simulink model "DAS"  (R2012b)
settings: Solver=FixedStepDiscrete  StartTime=0.0  StopTime=inf  FixedStep=0.1  RelTol=1e-3
PreLoadFcn:
  | if exist('tl_preloadfcn','file'), tl_preloadfcn(gcs,101); end
PostLoadFcn:
  | if exist('tl_postloadfcn','file'), tl_postloadfcn(gcs,101); end
InitFcn:
  | if exist('tlds_init','file'), tlds_init(gcs); end
StartFcn:
  | if exist('tlds_start','file'), tlds_start(gcs); end
StopFcn:
  | if exist('tlds_stop','file'), tlds_stop(gcs); end
undefined symbols (not defined in the file): A, B, C, Dd, DEMO_FAS_Accusti_Threshold_Time, DEMO_FAS_BrakeBooster_Threshold, DEMO_FAS_CC_DELTA, DEMO_FAS_CC_Lvl2_Round, DEMO_FAS_CC_Min_Value, DEMO_FAS_Distance_Treshold_Far, DEMO_FAS_Distance_Treshold_Med, DEMO_FAS_Distance_Treshold_Near, DEMO_FAS_Distronic, DEMO_FAS_Emerg_Brake_Force1, DEMO_FAS_Emerg_Brake_Force2, DEMO_FAS_Emerg_Brake_Time1, DEMO_FAS_Emerg_Brake_Time2, DEMO_FAS_EmergencyBrake, DEMO_FAS_FollowToStop, DEMO_FAS_Limiter, DEMO_FAS_Limiter_DELTA, DEMO_FAS_Neg_Max_ms, DEMO_FAS_Opti_Threshold_Time, DEMO_FAS_Repeater, DEMO_FAS_Repeater_Time, DEMO_FAS_Signdetection, DEMO_FAS_Tempomat
(part 7 of 11)

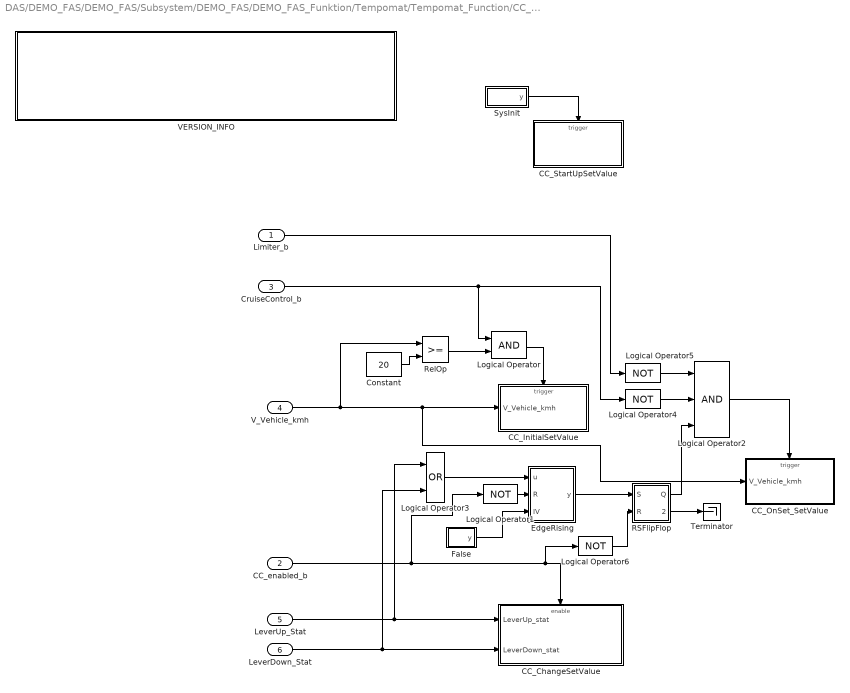
== system DAS/DEMO_FAS/DEMO_FAS/Subsystem/DEMO_FAS/DEMO_FAS_Funktion/Tempomat/Tempomat_Function/CC_SetValue ==
  Limiter_b : Inport
  CC_enabled_b : Inport  Port=2
  CruiseControl_b : Inport  Port=3
  V_Vehicle_kmh : Inport  Port=4
  LeverUp_Stat : Inport  Port=5
  LeverDown_Stat : Inport  Port=6
  CC_ChangeSetValue : Subsystem  TreatAsAtomicUnit=on
  CC_InitialSetValue : Subsystem  TreatAsAtomicUnit=on
  CC_OnSet_SetValue : Subsystem  TreatAsAtomicUnit=on
  CC_StartUpSetValue : Subsystem  TreatAsAtomicUnit=on
  Constant : Constant  Value=20  mask(TL_Constant){data={'date',735343.57031072921}}
      settings: CopyFcn=if exist('tl_reset_reviewflag') == 2, tl_reset_reviewflag(gcbh); end  DeleteFcn=if exist('delete_tlblock','file')==2,delete_tlblock(gcbh);end  NameChangeFcn=if exist('rename_tlblock','file')==2,rename_tlblock(gcbh);end  OpenFcn=if exist('tl_open_blockdlg','file')==2,tl_open_blockdlg(gcbh);else,open_system(gcbh,'parameter');end
      mask Help: eval(['if exist(''tl_online_help'',''file'') == 2, tl_online_help(''Topic'',''TL_Constant''),else, web([''jar:file:///'',matlabroot,''/help/toolbox/simulink/help.jar!/slref/' lower(get_param(gcbh,'Blocktype')) '.html''], ''-helpbrowser''),end'])
      mask Display: plot([-0.05, 1.05, NaN, -0.05, 1.05],[.01, .01, NaN, .99, .99])
  EdgeRising : Subsystem  mask(TLMSR_V200_EdgeRising){dT=-1, YName=}
      mask prompts: dT "Sampe Time"; YName "Y OutName"
      mask help:
      | The output indicates TRUE if the input value changes from FALSE to TRUE.
      | Reset input 'R' on TRUE will write the initial value 'IV' to the internal memory.
      mask init:
      | % TL block lines
      | x1=[0 0 1 1 0];
      | y1=[1 0 0 1 1];
      | x2=[1 0];
      | y2=[.96 .96];
      | x3=[0 1];
      | y3=[.04 .04];
      | 
      | tl_act_sg_init_blk;
      mask Help:
      | <HTML>
      | <HEAD>
      | <META HTTP-EQUIV="Content-Type" CONTENT="text/html; charset=iso-8859-1">
      | <TITLE>Help</TITLE>
      | </HEAD>
      | <BODY>
      | 
      | <B><FONT FACE="Arial"><P>Function:</P>
      | </B><P>The block detects a rising edge of the logical input signal <FONT FACE="Courier New">u</FONT> and indicates this change at the output <FONT FACE="Courier New">y</FONT> for one cycle.</P>
      | 
      | <B><P>In-/Outputs:</P>
      | </B>
      | <P><U>Input</U></P>
      | <P>The block input </FONT><FONT FACE="Courier New">u</FONT><FONT FACE="Arial"> must be connected to the input signal.</P>
      | 
      | <U><P>Reset / Initial Value</P>
      | </U><P>If the reset input </FONT><FONT FACE="Courier New">R</FONT><FONT FACE="Arial"> gets a '1' signal the block will write the initial value <FONT FACE="Courier New">IV</FONT> to its internal memory. A logical '1' at <FONT FACE="Courier New">IV</FONT>
      | will prevent the output to become TRUE during reset.</P>
      | 
      | <U><P>Output</P>
      | </U><P>The output </FONT><FONT FACE="Courier New">y</FONT><FONT FACE="Arial"> shows '1' if a rising edge at the input signal <FONT FACE="Courier New">u</FONT> is detected.</P>
      | </FONT></BODY>
      | </HTML>
      mask Display:
      | plot(x1,y1,x2,y2,x3,y3);
      | image(imread('EdgeRising.tif','tif'),[0.25,0.2,0.5,0.6])
  False : Subsystem  mask(TLACT_SG_V200_False){}
      mask help: False
      mask init:
      | % TL block lines
      | x1=[0 0 1 1 0];
      | y1=[1 0 0 1 1];
      | x2=[1 0];
      | y2=[.9 .9];
      | x3=[0 1];
      | y3=[.1 .1];
      settings: OpenFcn=open_system([gcb, '/Zero'], 'OpenFcn')
      mask Display:
      | plot(x1,y1,x2,y2,x3,y3);
      | disp('False');
  Logical Operator : Logic  AllPortsSameDT=off  OutDataTypeStr=boolean  mask(TL_LogicalOperator){data={'date',735343.57067486108}}
      settings: DeleteFcn=if exist('delete_tlblock','file')==2,delete_tlblock(gcbh);end  NameChangeFcn=if exist('rename_tlblock','file')==2,rename_tlblock(gcbh);end  OpenFcn=if exist('tl_open_blockdlg','file')==2,tl_open_blockdlg(gcbh);else,open_system(gcbh,'parameter');end
      mask Help: eval(['if exist(''tl_online_help'',''file'') == 2, tl_online_help(''Topic'',''TL_LogicalOperator''),else, web([''jar:file:///'',matlabroot,''/help/toolbox/simulink/help.jar!/slref/' lower(get_param(gcbh,'Blocktype')) '.html''], ''-helpbrowser''),end'])
      mask Display: plot([-0.05, 1.05, NaN, -0.05, 1.05],[.01, .01, NaN, .99, .99])
  Logical Operator{1,4..6} (4 alike) : Logic  Operator=NOT  Inputs=1  AllPortsSameDT=off  OutDataTypeStr=boolean  mask(TL_LogicalOperator){data={'date',735346.37280901615}}
      settings: DeleteFcn=if exist('delete_tlblock','file')==2,delete_tlblock(gcbh);end  NameChangeFcn=if exist('rename_tlblock','file')==2,rename_tlblock(gcbh);end  OpenFcn=if exist('tl_open_blockdlg','file')==2,tl_open_blockdlg(gcbh);else,open_system(gcbh,'parameter');end
      mask Help: eval(['if exist(''tl_online_help'',''file'') == 2, tl_online_help(''Topic'',''TL_LogicalOperator''),else, web([''jar:file:///'',matlabroot,''/help/toolbox/simulink/help.jar!/slref/' lower(get_param(gcbh,'Blocktype')) '.html''], ''-helpbrowser''),end'])
      mask Display: plot([-0.05, 1.05, NaN, -0.05, 1.05],[.01, .01, NaN, .99, .99])
  Logical Operator2 : Logic  Inputs=3  AllPortsSameDT=off  OutDataTypeStr=boolean  mask(TL_LogicalOperator){data={'date',735346.47148690966}}
      settings: DeleteFcn=if exist('delete_tlblock','file')==2,delete_tlblock(gcbh);end  NameChangeFcn=if exist('rename_tlblock','file')==2,rename_tlblock(gcbh);end  OpenFcn=if exist('tl_open_blockdlg','file')==2,tl_open_blockdlg(gcbh);else,open_system(gcbh,'parameter');end
      mask Help: eval(['if exist(''tl_online_help'',''file'') == 2, tl_online_help(''Topic'',''TL_LogicalOperator''),else, web([''jar:file:///'',matlabroot,''/help/toolbox/simulink/help.jar!/slref/' lower(get_param(gcbh,'Blocktype')) '.html''], ''-helpbrowser''),end'])
      mask Display: plot([-0.05, 1.05, NaN, -0.05, 1.05],[.01, .01, NaN, .99, .99])
  Logical Operator3 : Logic  Operator=OR  AllPortsSameDT=off  OutDataTypeStr=boolean  mask(TL_LogicalOperator){data={'date',735346.37234638887}}
      settings: DeleteFcn=if exist('delete_tlblock','file')==2,delete_tlblock(gcbh);end  NameChangeFcn=if exist('rename_tlblock','file')==2,rename_tlblock(gcbh);end  OpenFcn=if exist('tl_open_blockdlg','file')==2,tl_open_blockdlg(gcbh);else,open_system(gcbh,'parameter');end
      mask Help: eval(['if exist(''tl_online_help'',''file'') == 2, tl_online_help(''Topic'',''TL_LogicalOperator''),else, web([''jar:file:///'',matlabroot,''/help/toolbox/simulink/help.jar!/slref/' lower(get_param(gcbh,'Blocktype')) '.html''], ''-helpbrowser''),end'])
      mask Display: plot([-0.05, 1.05, NaN, -0.05, 1.05],[.01, .01, NaN, .99, .99])
  RSFlipFlop : Subsystem  mask(TLMSR_V200_RSFlipFlop){dT=-1, QName=, QNName=}
      mask prompts: dT "SampleTime"; QName "Q OutName"; QNName "QN OutName"
      mask help: A flip flop. The 'R' input (reset) dominates the 'S' input (set).
      mask init:
      | % TL block lines
      | x1=[0 0 1 1 0];
      | y1=[1 0 0 1 1];
      | x2=[1 0];
      | y2=[.96 .96];
      | x3=[0 1];
      | y3=[.04 .04];
      | 
      | tl_act_sg_init_blk;
      mask Help:
      | <HTML>
      | <HEAD>
      | <META HTTP-EQUIV="Content-Type" CONTENT="text/html; charset=iso-8859-1">
      | <TITLE>test</TITLE>
      | </HEAD>
      | 
      | <B><FONT FACE="Arial"><P>Function:</P>
      | </B><P>The block provides the function of a RS-Flip-Flop with the reset input </FONT><FONT FACE="Courier New">R</FONT><FONT FACE="Arial"> dominating over the set input </FONT><FONT FACE="Courier New">S</FONT><FONT FACE="Arial">. An inverted output </FONT><FONT FACE="Courier New">/Q</FONT><FONT FACE="Arial"> is provided.</P>
      | </FONT>
      | <TABLE BORDER CELLSPACING=1 CELLPADDING=4 WIDTH=506>
      | <TR><TD WIDTH="25%" VALIGN="TOP">
      | <B><FONT FACE="Arial"><P ALIGN="CENTER">S</B></FONT></TD>
      | <TD WIDTH="25%" VALIGN="TOP">
      | <B><FONT FACE="Arial"><P ALIGN="CENTER">R</B></FONT></TD>
      | <TD WIDTH="25%" VALIGN="TOP">
      | <B><FONT FACE="Arial"><P ALIGN="CENTER">Q</B></FONT></TD>
      | <TD WIDTH="25%" VALIGN="TOP">
      | <B><FONT FACE="Arial"><P ALIGN="CENTER">/Q</B></FONT></TD>
      | </TR>
      | <TR><TD WIDTH="25%" VALIGN="TOP">
      | <FONT FACE="Arial"><P ALIGN="CENTER">0</FONT></TD>
      | <TD WIDTH="25%" VALIGN="TOP">
      | <FONT FACE="Arial"><P ALIGN="CENTER">0</FONT></TD>
      | <TD WIDTH="25%" VALIGN="TOP">
      | <FONT FACE="Arial"><P ALIGN="CENTER">Q(n-1)</FONT></TD>
      | <TD WIDTH="25%" VALIGN="TOP">
      | <FONT FACE="Arial"><P ALIGN="CENTER">/Q(n-1)</FONT></TD>
      | </TR>
      | <TR><TD WIDTH="25%" VALIGN="TOP">
      | <FONT FACE="Arial"><P ALIGN="CENTER">0</FONT></TD>
      | <TD WIDTH="25%" VALIGN="TOP">
      | <FONT FACE="Arial"><P ALIGN="CENTER">1</FONT></TD>
      | <TD WIDTH="25%" VALIGN="TOP">
      | <FONT FACE="Arial"><P ALIGN="CENTER">0</FONT></TD>
      | <TD WIDTH="25%" VALIGN="TOP">
      | <FONT FACE="Arial"><P ALIGN="CENTER">1</FONT></TD>
      | </TR>
      | <TR><TD WIDTH="25%" VALIGN="TOP">
      | <FONT FACE="Arial"><P ALIGN="CENTER">1</FONT></TD>
      | <TD WIDTH="25%" VALIGN="TOP">
      | <FONT FACE="Arial"><P ALIGN="CENTER">0</FONT></TD>
      | <TD WIDTH="25%" VALIGN="TOP">
      | <FONT FACE="Arial"><P ALIGN="CENTER">1</FONT></TD>
      | <TD WIDTH="25%" VALIGN="TOP">
      | <FONT FACE="Arial"><P ALIGN="CENTER">0</FONT></TD>
      | </TR>
      | <TR><TD WIDTH="25%" VALIGN="TOP">
      | <FONT FACE="Arial"><P ALIGN="CENTER">1</FONT></TD>
      | <TD WIDTH="25%" VALIGN="TOP">
      | <FONT FACE="Arial"><P ALIGN="CENTER">1</FONT></TD>
      | <TD WIDTH="25%" VALIGN="TOP">
      | <FONT FACE="Arial"><P ALIGN="CENTER">0</FONT></TD>
      | <TD WIDTH="25%" VALIGN="TOP">
      | <FONT FACE="Arial"><P ALIGN="CENTER">1</FONT></TD>
      | </TR>
      | </TABLE>
      | 
      | <FONT FACE="Arial">
      | <B><P>In-/Outputs:</P>
      | </B><U><P>S</P>
      | </U><P>The set input </FONT><FONT FACE="Courier New">S</FONT><FONT FACE="Arial"> on '1' will set the output </FONT><FONT FACE="Courier New">Q</FONT><FONT FACE="Arial"> if the reset input </FONT><FONT FACE="Courier New">R</FONT><FONT FACE="Arial"> is '0'.</P>
      | <U><P>R</P>
      | </U><P>The reset input </FONT><FONT FACE="Courier New">R</FONT><FONT FACE="Arial"> on '1' will reset the output </FONT><FONT FACE="Courier New">Q</FONT><FONT FACE="Arial">.</P>
      | <U><P>Q, /Q</P>
      | </U><P>The output </FONT><FONT FACE="Courier New">Q</FONT><FONT FACE="Arial"> shows the state of the internal memory. </FONT><FONT FACE="Courier New">/Q</FONT><FONT FACE="Arial"> contains the inverted state of </FONT><FONT FACE="Courier New">Q</FONT><FONT FACE="Arial">.</P></FONT>
      | </HTML>
      mask Display:
      | plot(x1,y1,x2,y2,x3,y3);
      | image(imread('RSFlipFlop.tif','tif'),[0.05,0.1,0.9,0.8])
  RelOp : RelationalOperator  Description=|  mask(TL_RelationalOperator){data={'logdata',{'plotchannels',[]},'date',735343.572069132}}
      | Relational operator block of dSPACE TargetLink.
      | 
      | This block performs a relational operation on its two inputs u1 and u2 and produces output according to the following table.
      | If the result is TRUE, the output is 1; if FALSE, it is 0.
      | 
      | Operator   Output
      |  ==        TRUE if u1 is equal to u2
      |  !=        TRUE if u1 is not equal to u2
      |  <         TRUE if u1 is less than u2
      |  <=        TRUE if u1 is less than or equal to u2
      |  >=        TRUE if u1 is greater than or equal to u2
      |  >         TRUE if u1 is greater than u2
      settings: DeleteFcn=if exist('delete_tlblock','file')==2,delete_tlblock(gcbh);end  NameChangeFcn=if exist('rename_tlblock','file')==2,rename_tlblock(gcbh);end  OpenFcn=if exist('tl_open_blockdlg','file')==2,tl_open_blockdlg(gcbh);else,open_system(gcbh,'parameter');end
      mask Help: eval(['if exist(''tl_online_help'',''file'') == 2, tl_online_help(''Topic'',''TL_RelationalOperator''),else, web([''jar:file:///'',matlabroot,''/help/toolbox/simulink/help.jar!/slref/' lower(get_param(gcbh,'Blocktype')) '.html''], ''-helpbrowser''),end'])
      mask Display: plot([-0.05, 1.05, NaN, -0.05, 1.05],[.01, .01, NaN, .99, .99])
  SysInit : Subsystem  mask(TLACT_SG_V200_SysInit){dT=-1, YName=}
      mask prompts: dT "Sample Time"; YName "Y OutName"
      mask help: An inital pulse is generated for for the first block evaluation.
      mask init:
      | % TL block lines
      | x1=[0 0 1 1 0];
      | y1=[1 0 0 1 1];
      | x2=[1 0];
      | y2=[.92 .92];
      | x3=[0 1];
      | y3=[.08 .08];
      | 
      | tl_act_sg_init_blk;
      mask Help:
      | <P><B>Function:</B></P>
      | <P>The block provides an initial pulse at the output on the first
      | evaluation of the block.<BR> This function can be used for system startup functions to
      | get defined states in the system.</P>
      | 
      | <P><B>In-/Outputs:</B></P>
      | <P><U>Output</U></P>
      | <P>The output shows TRUE at the first cycle, else it shows FALSE.</P>
      mask Display:
      | plot(x1,y1,x2,y2,x3,y3);
      | disp('SysInit');
  Terminator : Terminator
  VERSION_INFO : Subsystem  mask(VERSION_INFO_BLOCK){versinfo_data=struct('modname','DEMO_FAS/DEMO_FAS_Funktion/Tempomat/Tempomat_Function/CC_SetValue','version','1.1.1','date','22-Apr-2013','author','YVEDUHR','modtype',3,'variant',0,'remark',{{'~'}},'copyright',['Daimler AG'],'SGMLdescr','','prefix','','pfx_act',0,'ntselect',3,'asize',0), versinfo_string=Model: DEMO_FAS/DEMO_FAS_Funktion/Tempomat/Tempomat_Function/CC_SetValue\nVersion: 1.1.1\nDate: 22-Apr-2013\nAuthor: YVEDUHR\nModule: INTERNAL\n\nAll copyrights by Daimler AG}
      mask prompts: versinfo_data "Mask Parameter 1"; versinfo_string "Mask Parameter 2"
      mask help:
      | This is a Version Info Subsystem (empty)
      | All version Information is stored in Parameter "versinfo_data" and displayed
      settings: OpenFcn=edit_subsys_info('init')
      mask Display: disp(versinfo_string);
  wires:
  SysInit/1(y) -> CC_StartUpSetValue/Trigger
  V_Vehicle_kmh/1 -> RelOp/1, CC_OnSet_SetValue/1(V_Vehicle_kmh), CC_InitialSetValue/1(V_Vehicle_kmh)
  Constant/1 -> RelOp/2
  RelOp/1 -> Logical Operator/2
  Logical Operator/1 -> CC_InitialSetValue/Trigger
  CruiseControl_b/1 -> Logical Operator4/1, Logical Operator/1
  LeverUp_Stat/1 -> Logical Operator3/1, CC_ChangeSetValue/1(LeverUp_stat)
  LeverDown_Stat/1 -> Logical Operator3/2, CC_ChangeSetValue/2(LeverDown_stat)
  CC_enabled_b/1 -> Logical Operator1/1, Logical Operator6/1, CC_ChangeSetValue/Enable
  Logical Operator3/1 -> EdgeRising/1(u)
  False/1(y) -> EdgeRising/3(IV)
  Logical Operator1/1 -> EdgeRising/2(R)
  Logical Operator2/1 -> CC_OnSet_SetValue/Trigger
  Logical Operator4/1 -> Logical Operator2/2
  EdgeRising/1(y) -> RSFlipFlop/1(S)
  Limiter_b/1 -> Logical Operator5/1
  Logical Operator5/1 -> Logical Operator2/1
  Logical Operator6/1 -> RSFlipFlop/2(R)
  RSFlipFlop/1(Q) -> Logical Operator2/3
  RSFlipFlop/2(NOT_Q) -> Terminator/1

== system DAS/DEMO_FAS/DEMO_FAS/Subsystem/DEMO_FAS/DEMO_FAS_Funktion/Tempomat/Tempomat_Function/VERSION_INFO ==
  Copyright : Subsystem
      mask help: Copyright
      mask Display: disp('All copyrights by DaimlerChrysler');

== system DAS/DEMO_FAS/DEMO_FAS/Subsystem/DEMO_FAS/DEMO_FAS_Funktion/Tempomat/VERSION_INFO/Copyright ==

== system DAS/DEMO_FAS/DEMO_FAS/Subsystem/DEMO_FAS/DEMO_FAS_Funktion/Velocity Control/VERSION_INFO/Copyright ==

== system DAS/DEMO_FAS/DEMO_FAS/Subsystem/DEMO_FAS/DEMO_FAS_Funktion/BrakeAssistant/Brake_Booster/VERSION_INFO/Copyright ==

== system DAS/DEMO_FAS/DEMO_FAS/Subsystem/DEMO_FAS/DEMO_FAS_Funktion/Distancewarner/Distancewarner_Function/VERSION_INFO/Copyright ==

== system DAS/DEMO_FAS/DEMO_FAS/Subsystem/DEMO_FAS/DEMO_FAS_Funktion/Distronic/Distronic_Deactive/VERSION_INFO/Copyright ==

== system DAS/DEMO_FAS/DEMO_FAS/Subsystem/DEMO_FAS/DEMO_FAS_Funktion/Distronic/Distronic_Disabled/VERSION_INFO/Copyright ==

== system DAS/DEMO_FAS/DEMO_FAS/Subsystem/DEMO_FAS/DEMO_FAS_Funktion/Distronic/Distronic_Enabled/VERSION_INFO/Copyright ==

== system DAS/DEMO_FAS/DEMO_FAS/Subsystem/DEMO_FAS/DEMO_FAS_Funktion/Distronic/Distronic_FTS_Enabled/VERSION_INFO/Copyright ==

== system DAS/DEMO_FAS/DEMO_FAS/Subsystem/DEMO_FAS/DEMO_FAS_Funktion/EmergencyBrake/EmergencyBrake_Function/VERSION_INFO/Copyright ==

== system DAS/DEMO_FAS/DEMO_FAS/Subsystem/DEMO_FAS/DEMO_FAS_Funktion/FollowToStop/FollowToStop_Function/VERSION_INFO/Copyright ==

== system DAS/DEMO_FAS/DEMO_FAS/Subsystem/DEMO_FAS/DEMO_FAS_Funktion/Limiter/Limiter_Function/Limiter_Enabled/EdgeRising ==
  u : Inport
  R : Inport  Port=2
  IV : Inport  Port=3
  LogOp_A : Logic  Description=|  AllPortsSameDT=off  mask(TL_LogicalOperator){data={'logdata',{'plotchannels',[]},'date',734383.73416157404}}
      | Logical operator block of dSPACE TargetLink.
      | 
      | The Logical Operator block performs any of these logical operations on its inputs: AND, OR, NAND, NOR, XOR, and NOT. A nonzero input is treated as TRUE (1), a zero input as FALSE (0). The output depends on the selected operator. The output is 1 if TRUE and 0 if FALSE.
      settings: DeleteFcn=if exist('delete_tlblock','file')==2,delete_tlblock(gcbh);end  NameChangeFcn=if exist('rename_tlblock','file')==2,rename_tlblock(gcbh);end  OpenFcn=if exist('tl_open_blockdlg','file')==2,tl_open_blockdlg(gcbh);else,open_system(gcbh,'parameter');end
      mask Help: eval(['if exist(''tl_online_help'',''file'') == 2, tl_online_help(''Topic'',''TL_LogicalOperator''),else, web([''jar:file:///'',matlabroot,''/help/toolbox/simulink/help.jar!/slref/' lower(get_param(gcbh,'Blocktype')) '.html''], ''-helpbrowser''),end'])
      mask Display: plot([-0.05, 1.05, NaN, -0.05, 1.05],[.01, .01, NaN, .99, .99])
  LogOp_N : Logic  Description=|  Operator=NOT  Inputs=1  AllPortsSameDT=off  mask(TL_LogicalOperator){data={'logdata',{'plotchannels',[]},'date',734383.73416121525}}
      | Logical operator block of dSPACE TargetLink.
      | 
      | The Logical Operator block performs any of these logical operations on its inputs: AND, OR, NAND, NOR, XOR, and NOT. A nonzero input is treated as TRUE (1), a zero input as FALSE (0). The output depends on the selected operator. The output is 1 if TRUE and 0 if FALSE.
      settings: DeleteFcn=if exist('delete_tlblock','file')==2,delete_tlblock(gcbh);end  NameChangeFcn=if exist('rename_tlblock','file')==2,rename_tlblock(gcbh);end  OpenFcn=if exist('tl_open_blockdlg','file')==2,tl_open_blockdlg(gcbh);else,open_system(gcbh,'parameter');end
      mask Help: eval(['if exist(''tl_online_help'',''file'') == 2, tl_online_help(''Topic'',''TL_LogicalOperator''),else, web([''jar:file:///'',matlabroot,''/help/toolbox/simulink/help.jar!/slref/' lower(get_param(gcbh,'Blocktype')) '.html''], ''-helpbrowser''),end'])
      mask Display: plot([-0.05, 1.05, NaN, -0.05, 1.05],[.01, .01, NaN, .99, .99])
  Memory_U : UnitDelay  Description=|  SampleTime=dT  mask(TL_UnitDelay){data={'logdata',{'plotchannels',[]},'output',{'type','Bool'},'state',{'type','Bool'},'date',734383.73416067124}}
      | Unit Delay block of dSPACE TargetLink.
      | 
      | Output signal is equal to the input signal of the last sample step:
      | 
      |         y(k) = u(k-1).
      | 
      | In the 1st sampling step, the output signal is initialized with 'initial condition':
      | 
      |         y(0) = initial condition
      settings: CopyFcn=if exist('tl_reset_reviewflag') == 2, tl_reset_reviewflag(gcbh); end  DeleteFcn=if exist('delete_tlblock','file')==2,delete_tlblock(gcbh);end  NameChangeFcn=if exist('rename_tlblock','file')==2,rename_tlblock(gcbh);end  OpenFcn=if exist('tl_open_blockdlg','file')==2,tl_open_blockdlg(gcbh);else,open_system(gcbh,'parameter');end
      mask Help: eval(['if exist(''tl_online_help'',''file'') == 2, tl_online_help(''Topic'',''TL_UnitDelay''),else, web([''jar:file:///'',matlabroot,''/help/toolbox/simulink/help.jar!/slref/' lower(get_param(gcbh,'Blocktype')) '.html''], ''-helpbrowser''),end'])
      mask Display: plot([-0.05, 1.05, NaN, -0.05, 1.05],[.01, .01, NaN, .99, .99])
  Switch_R : Switch  Description=|  Threshold=1  mask(TL_Switch){data={'logdata',{'plotchannels',[]},'output',{'type','Bool'},'date',734383.73415995366}}
      | Switch block of dSPACE TargetLink.
      | 
      | Passes through input 1 if input 2 is greater than or equal to threshold, otherwise, passes through input 3:
      | 
      | if u2 >= threshold
      |    y = u1;
      | else
      |    y = u3;
      | end
      settings: CopyFcn=if exist('tl_reset_reviewflag') == 2, tl_reset_reviewflag(gcbh); end  DeleteFcn=if exist('delete_tlblock','file')==2,delete_tlblock(gcbh);end  NameChangeFcn=if exist('rename_tlblock','file')==2,rename_tlblock(gcbh);end  OpenFcn=if exist('tl_open_blockdlg','file')==2,tl_open_blockdlg(gcbh);else,open_system(gcbh,'parameter');end
      mask Help: eval(['if exist(''tl_online_help'',''file'') == 2, tl_online_help(''Topic'',''TL_Switch''),else, web([''jar:file:///'',matlabroot,''/help/toolbox/simulink/help.jar!/slref/' lower(get_param(gcbh,'Blocktype')) '.html''], ''-helpbrowser''),end'])
      mask Display: plot([-0.05, 1.05, NaN, -0.05, 1.05],[.01, .01, NaN, .99, .99])
  y : Outport  InitialOutput=0
  wires:
  IV/1 -> Switch_R/1
  Memory_U/1 -> Switch_R/3
  R/1 -> Switch_R/2
  Switch_R/1 -> LogOp_N/1
  u/1 -> Memory_U/1, LogOp_A/1
  LogOp_A/1 -> y/1
  LogOp_N/1 -> LogOp_A/2

== system DAS/DEMO_FAS/DEMO_FAS/Subsystem/DEMO_FAS/DEMO_FAS_Funktion/Limiter/Limiter_Function/Limiter_Enabled/False ==
  Zero : Constant  Description=|  Value=0  SampleTime=-1  mask(TL_Constant){data={'output',{'tolerance',0},'date',734383.73403155094}}
      | Constant block of dSPACE TargetLink.
      | 
      | Output signal keeps the given constant value.
      settings: DeleteFcn=if exist('delete_tlblock','file')==2,delete_tlblock(gcbh);end  NameChangeFcn=if exist('rename_tlblock','file')==2,rename_tlblock(gcbh);end  OpenFcn=if exist('tl_open_blockdlg','file')==2,tl_open_blockdlg(gcbh);else,open_system(gcbh,'parameter');end
      mask Help: eval(['if exist(''tl_online_help'',''file'') == 2, tl_online_help(''Topic'',''TL_Constant''),else, web([''jar:file:///'',matlabroot,''/help/toolbox/simulink/help.jar!/slref/' lower(get_param(gcbh,'Blocktype')) '.html''], ''-helpbrowser''),end'])
      mask Display: plot([-0.05, 1.05, NaN, -0.05, 1.05],[.01, .01, NaN, .99, .99])
  y : Outport
  wires:
  Zero/1 -> y/1

== system DAS/DEMO_FAS/DEMO_FAS/Subsystem/DEMO_FAS/DEMO_FAS_Funktion/Limiter/Limiter_Function/Limiter_Enabled/Limiter_Active ==
  Action Port : ActionPort  ActionType=then
  Data Store Read1 : DataStoreRead  Description=|  DataStoreName=DEMO_FAS_V_LimiterSetValue  mask(TL_DataStoreRead){data={'logdata',{'plotchannels',[]},'date',735342.52721385413}}
      | Data Store Read block of dSPACE TargetLink.
      | Use this block to specify inputs from global variables within the production code application.
      settings: DeleteFcn=if exist('delete_tlblock','file')==2,delete_tlblock(gcbh);end  NameChangeFcn=if exist('rename_tlblock','file')==2,rename_tlblock(gcbh);end  OpenFcn=if exist('tl_open_blockdlg','file')==2,tl_open_blockdlg(gcbh);else,open_system(gcbh,'parameter');end
      mask Help: eval(['if exist(''tl_online_help'',''file'') == 2, tl_online_help(''Topic'',''TL_DataStoreRead''),else, web([''jar:file:///'',matlabroot,''/help/toolbox/simulink/help.jar!/slref/' lower(get_param(gcbh,'Blocktype')) '.html''], ''-helpbrowser''),end'])
      mask Display: plot([-0.05, 1.05, NaN, -0.05, 1.05],[.01, .01, NaN, .99, .99])
  Gain : Gain  Description=|  mask(TL_Gain){data={'logdata',{'plotchannels',[]},'date',734383.73388723377}}
      | Gain block of dSPACE TargetLink.
      | 
      | Output signal is equal to the product of the input signal and the gain value:
      |         y = G u
      settings: CopyFcn=if exist('tl_reset_reviewflag') == 2, tl_reset_reviewflag(gcbh); end  DeleteFcn=if exist('delete_tlblock','file')==2,delete_tlblock(gcbh);end  NameChangeFcn=if exist('rename_tlblock','file')==2,rename_tlblock(gcbh);end  OpenFcn=if exist('tl_open_blockdlg','file')==2,tl_open_blockdlg(gcbh);else,open_system(gcbh,'parameter');end
      mask Help: eval(['if exist(''tl_online_help'',''file'') == 2, tl_online_help(''Topic'',''TL_Gain''),else, web([''jar:file:///'',matlabroot,''/help/toolbox/simulink/help.jar!/slref/' lower(get_param(gcbh,'Blocktype')) '.html''], ''-helpbrowser''),end'])
      mask Display: plot([0, .9, 0],[.05, .5, .95])
  Logical Operator : Logic  AllPortsSameDT=off  OutDataTypeStr=boolean  mask(TL_LogicalOperator){data={'date',735360.45292877313}}
      settings: DeleteFcn=if exist('delete_tlblock','file')==2,delete_tlblock(gcbh);end  NameChangeFcn=if exist('rename_tlblock','file')==2,rename_tlblock(gcbh);end  OpenFcn=if exist('tl_open_blockdlg','file')==2,tl_open_blockdlg(gcbh);else,open_system(gcbh,'parameter');end
      mask Help: eval(['if exist(''tl_online_help'',''file'') == 2, tl_online_help(''Topic'',''TL_LogicalOperator''),else, web([''jar:file:///'',matlabroot,''/help/toolbox/simulink/help.jar!/slref/' lower(get_param(gcbh,'Blocktype')) '.html''], ''-helpbrowser''),end'])
      mask Display: plot([-0.05, 1.05, NaN, -0.05, 1.05],[.01, .01, NaN, .99, .99])
  True : Subsystem  mask(TLACT_SG_V200_True){}
      mask help: True
      mask init:
      | % TL block lines
      | x1=[0 0 1 1 0];
      | y1=[1 0 0 1 1];
      | x2=[1 0];
      | y2=[.9 .9];
      | x3=[0 1];
      | y3=[.1 .1];
      settings: OpenFcn=open_system([gcb, '/One'], 'OpenFcn')
      mask Display:
      | plot(x1,y1,x2,y2,x3,y3);
      | disp('True')
  VERSION_INFO : Subsystem  mask(VERSION_INFO_BLOCK){versinfo_data=struct('modname','DEMO_FAS/DEMO_FAS_Funktion/Limiter/Limiter_Function/Limiter_Enabled/Limiter_Active','version','1.1.1','date','18-Apr-2013','author','YVEDUHR','modtype',3,'variant',0,'remark',{{'~'}},'copyright',['Daimler AG'],'SGMLdescr','','prefix','','pfx_act',0,'ntselect',3,'asize',0), versinfo_string=Model: DEMO_FAS/DEMO_FAS_Funktion/Limiter/Limiter_Function/Limiter_Enabled/Limiter_Active\nVersion: 1.1.1\nDate: 18-Apr-2013\nAuthor: YVEDUHR\nModule: INTERNAL\n\nAll copyrights by Daimler AG}
      mask prompts: versinfo_data "Mask Parameter 1"; versinfo_string "Mask Parameter 2"
      mask help:
      | This is a Version Info Subsystem (empty)
      | All version Information is stored in Parameter "versinfo_data" and displayed
      settings: OpenFcn=edit_subsys_info('init')
      mask Display: disp(versinfo_string);
  VMax_kmh : Outport
  Limiter_active_b : Outport  Port=2  InitialOutput=0
  wires:
  Data Store Read1/1 -> Gain/1  "VMax_kmh"
  True/1(y) -> Logical Operator/2, Logical Operator/1  "Limiter_enabled_b"
  Logical Operator/1 -> Limiter_active_b/1  "Limiter_active_b"
  Gain/1 -> VMax_kmh/1  "VMax_kmh"

== system DAS/DEMO_FAS/DEMO_FAS/Subsystem/DEMO_FAS/DEMO_FAS_Funktion/Limiter/Limiter_Function/Limiter_Enabled/Limiter_Deactive ==
  Action Port : ActionPort  ActionType=else
  Constant : Constant  Value=300  mask(TL_Constant){data={'date',735339.6921373033}}
      settings: CopyFcn=if exist('tl_reset_reviewflag') == 2, tl_reset_reviewflag(gcbh); end  DeleteFcn=if exist('delete_tlblock','file')==2,delete_tlblock(gcbh);end  NameChangeFcn=if exist('rename_tlblock','file')==2,rename_tlblock(gcbh);end  OpenFcn=if exist('tl_open_blockdlg','file')==2,tl_open_blockdlg(gcbh);else,open_system(gcbh,'parameter');end
      mask Help: eval(['if exist(''tl_online_help'',''file'') == 2, tl_online_help(''Topic'',''TL_Constant''),else, web([''jar:file:///'',matlabroot,''/help/toolbox/simulink/help.jar!/slref/' lower(get_param(gcbh,'Blocktype')) '.html''], ''-helpbrowser''),end'])
      mask Display: plot([-0.05, 1.05, NaN, -0.05, 1.05],[.01, .01, NaN, .99, .99])
  False : Subsystem  mask(TLACT_SG_V200_False){}
      mask help: False
      mask init:
      | % TL block lines
      | x1=[0 0 1 1 0];
      | y1=[1 0 0 1 1];
      | x2=[1 0];
      | y2=[.9 .9];
      | x3=[0 1];
      | y3=[.1 .1];
      settings: OpenFcn=open_system([gcb, '/Zero'], 'OpenFcn')
      mask Display:
      | plot(x1,y1,x2,y2,x3,y3);
      | disp('False');
  Gain : Gain  Description=|  mask(TL_Gain){data={'logdata',{'plotchannels',[]},'date',734383.73388723377}}
      | Gain block of dSPACE TargetLink.
      | 
      | Output signal is equal to the product of the input signal and the gain value:
      |         y = G u
      settings: CopyFcn=if exist('tl_reset_reviewflag') == 2, tl_reset_reviewflag(gcbh); end  DeleteFcn=if exist('delete_tlblock','file')==2,delete_tlblock(gcbh);end  NameChangeFcn=if exist('rename_tlblock','file')==2,rename_tlblock(gcbh);end  OpenFcn=if exist('tl_open_blockdlg','file')==2,tl_open_blockdlg(gcbh);else,open_system(gcbh,'parameter');end
      mask Help: eval(['if exist(''tl_online_help'',''file'') == 2, tl_online_help(''Topic'',''TL_Gain''),else, web([''jar:file:///'',matlabroot,''/help/toolbox/simulink/help.jar!/slref/' lower(get_param(gcbh,'Blocktype')) '.html''], ''-helpbrowser''),end'])
      mask Display: plot([0, .9, 0],[.05, .5, .95])
  Logical Operator : Logic  AllPortsSameDT=off  OutDataTypeStr=boolean  mask(TL_LogicalOperator){data={'date',735360.45292877313}}
      settings: DeleteFcn=if exist('delete_tlblock','file')==2,delete_tlblock(gcbh);end  NameChangeFcn=if exist('rename_tlblock','file')==2,rename_tlblock(gcbh);end  OpenFcn=if exist('tl_open_blockdlg','file')==2,tl_open_blockdlg(gcbh);else,open_system(gcbh,'parameter');end
      mask Help: eval(['if exist(''tl_online_help'',''file'') == 2, tl_online_help(''Topic'',''TL_LogicalOperator''),else, web([''jar:file:///'',matlabroot,''/help/toolbox/simulink/help.jar!/slref/' lower(get_param(gcbh,'Blocktype')) '.html''], ''-helpbrowser''),end'])
      mask Display: plot([-0.05, 1.05, NaN, -0.05, 1.05],[.01, .01, NaN, .99, .99])
  VERSION_INFO : Subsystem  mask(VERSION_INFO_BLOCK){versinfo_data=struct('modname','DEMO_FAS/DEMO_FAS_Funktion/Limiter/Limiter_Function/Limiter_Enabled/Limiter_Deactive','version','1.1.1','date','18-Apr-2013','author','YVEDUHR','modtype',3,'variant',0,'remark',{{'~'}},'copyright',['Daimler AG'],'SGMLdescr','','prefix','','pfx_act',0,'ntselect',3,'asize',0), versinfo_string=Model: DEMO_FAS/DEMO_FAS_Funktion/Limiter/Limiter_Function/Limiter_Enabled/Limiter_Deactive\nVersion: 1.1.1\nDate: 18-Apr-2013\nAuthor: YVEDUHR\nModule: INTERNAL\n\nAll copyrights by Daimler AG}
      mask prompts: versinfo_data "Mask Parameter 1"; versinfo_string "Mask Parameter 2"
      mask help:
      | This is a Version Info Subsystem (empty)
      | All version Information is stored in Parameter "versinfo_data" and displayed
      settings: OpenFcn=edit_subsys_info('init')
      mask Display: disp(versinfo_string);
  VMax_kmh : Outport  InitialOutput=300
  Limiter_active_b : Outport  Port=2  InitialOutput=0
  wires:
  False/1(y) -> Logical Operator/1, Logical Operator/2  "Limiter_active_b"
  Constant/1 -> Gain/1  "VMax_kmh"
  Logical Operator/1 -> Limiter_active_b/1  "Limiter_active_b"
  Gain/1 -> VMax_kmh/1  "VMax_kmh"

== system DAS/DEMO_FAS/DEMO_FAS/Subsystem/DEMO_FAS/DEMO_FAS_Funktion/Limiter/Limiter_Function/Limiter_Enabled/RSFlipFlop ==
  S : Inport
  R : Inport  Port=2
  LogOp_N : Logic  Description=|  Operator=NOT  Inputs=1  AllPortsSameDT=off  mask(TL_LogicalOperator){data={'logdata',{'plotchannels',[]},'date',734383.73415922455}}
      | Logical operator block of dSPACE TargetLink.
      | 
      | The Logical Operator block performs any of these logical operations on its inputs: AND, OR, NAND, NOR, XOR, and NOT. A nonzero input is treated as TRUE (1), a zero input as FALSE (0). The output depends on the selected operator. The output is 1 if TRUE and 0 if FALSE.
      settings: DeleteFcn=if exist('delete_tlblock','file')==2,delete_tlblock(gcbh);end  NameChangeFcn=if exist('rename_tlblock','file')==2,rename_tlblock(gcbh);end  OpenFcn=if exist('tl_open_blockdlg','file')==2,tl_open_blockdlg(gcbh);else,open_system(gcbh,'parameter');end
      mask Help: eval(['if exist(''tl_online_help'',''file'') == 2, tl_online_help(''Topic'',''TL_LogicalOperator''),else, web([''jar:file:///'',matlabroot,''/help/toolbox/simulink/help.jar!/slref/' lower(get_param(gcbh,'Blocktype')) '.html''], ''-helpbrowser''),end'])
      mask Display: plot([-0.05, 1.05, NaN, -0.05, 1.05],[.01, .01, NaN, .99, .99])
  Memory_Q : UnitDelay  Description=|  SampleTime=dT  mask(TL_UnitDelay){data={'logdata',{'plotchannels',[]},'output',{'type','Bool'},'state',{'type','Bool'},'date',734383.73415886576}}
      | Unit Delay block of dSPACE TargetLink.
      | 
      | Output signal is equal to the input signal of the last sample step:
      | 
      |         y(k) = u(k-1).
      | 
      | In the 1st sampling step, the output signal is initialized with 'initial condition':
      | 
      |         y(0) = initial condition
      settings: CopyFcn=if exist('tl_reset_reviewflag') == 2, tl_reset_reviewflag(gcbh); end  DeleteFcn=if exist('delete_tlblock','file')==2,delete_tlblock(gcbh);end  NameChangeFcn=if exist('rename_tlblock','file')==2,rename_tlblock(gcbh);end  OpenFcn=if exist('tl_open_blockdlg','file')==2,tl_open_blockdlg(gcbh);else,open_system(gcbh,'parameter');end
      mask Help: eval(['if exist(''tl_online_help'',''file'') == 2, tl_online_help(''Topic'',''TL_UnitDelay''),else, web([''jar:file:///'',matlabroot,''/help/toolbox/simulink/help.jar!/slref/' lower(get_param(gcbh,'Blocktype')) '.html''], ''-helpbrowser''),end'])
      mask Display: plot([-0.05, 1.05, NaN, -0.05, 1.05],[.01, .01, NaN, .99, .99])
  One_S : Constant  Description=|  mask(TL_Constant){data={'date',734383.73415796296}}
      | Constant block of dSPACE TargetLink.
      | 
      | Output signal keeps the given constant value.
      settings: DeleteFcn=if exist('delete_tlblock','file')==2,delete_tlblock(gcbh);end  NameChangeFcn=if exist('rename_tlblock','file')==2,rename_tlblock(gcbh);end  OpenFcn=if exist('tl_open_blockdlg','file')==2,tl_open_blockdlg(gcbh);else,open_system(gcbh,'parameter');end
      mask Help: eval(['if exist(''tl_online_help'',''file'') == 2, tl_online_help(''Topic'',''TL_Constant''),else, web([''jar:file:///'',matlabroot,''/help/toolbox/simulink/help.jar!/slref/' lower(get_param(gcbh,'Blocktype')) '.html''], ''-helpbrowser''),end'])
      mask Display: plot([-0.05, 1.05, NaN, -0.05, 1.05],[.01, .01, NaN, .99, .99])
  Switch_R : Switch  Description=|  Threshold=1  mask(TL_Switch){data={'logdata',{'plotchannels',[]},'output',{'type','Bool'},'date',734383.73415760417}}
      | Switch block of dSPACE TargetLink.
      | 
      | Passes through input 1 if input 2 is greater than or equal to threshold, otherwise, passes through input 3:
      | 
      | if u2 >= threshold
      |    y = u1;
      | else
      |    y = u3;
      | end
      settings: CopyFcn=if exist('tl_reset_reviewflag') == 2, tl_reset_reviewflag(gcbh); end  DeleteFcn=if exist('delete_tlblock','file')==2,delete_tlblock(gcbh);end  NameChangeFcn=if exist('rename_tlblock','file')==2,rename_tlblock(gcbh);end  OpenFcn=if exist('tl_open_blockdlg','file')==2,tl_open_blockdlg(gcbh);else,open_system(gcbh,'parameter');end
      mask Help: eval(['if exist(''tl_online_help'',''file'') == 2, tl_online_help(''Topic'',''TL_Switch''),else, web([''jar:file:///'',matlabroot,''/help/toolbox/simulink/help.jar!/slref/' lower(get_param(gcbh,'Blocktype')) '.html''], ''-helpbrowser''),end'])
      mask Display: plot([-0.05, 1.05, NaN, -0.05, 1.05],[.01, .01, NaN, .99, .99])
  Switch_S : Switch  Description=|  Threshold=1  mask(TL_Switch){data={'logdata',{'plotchannels',[]},'output',{'type','Bool'},'date',734383.73415668984}}
      | Switch block of dSPACE TargetLink.
      | 
      | Passes through input 1 if input 2 is greater than or equal to threshold, otherwise, passes through input 3:
      | 
      | if u2 >= threshold
      |    y = u1;
      | else
      |    y = u3;
      | end
      settings: CopyFcn=if exist('tl_reset_reviewflag') == 2, tl_reset_reviewflag(gcbh); end  DeleteFcn=if exist('delete_tlblock','file')==2,delete_tlblock(gcbh);end  NameChangeFcn=if exist('rename_tlblock','file')==2,rename_tlblock(gcbh);end  OpenFcn=if exist('tl_open_blockdlg','file')==2,tl_open_blockdlg(gcbh);else,open_system(gcbh,'parameter');end
      mask Help: eval(['if exist(''tl_online_help'',''file'') == 2, tl_online_help(''Topic'',''TL_Switch''),else, web([''jar:file:///'',matlabroot,''/help/toolbox/simulink/help.jar!/slref/' lower(get_param(gcbh,'Blocktype')) '.html''], ''-helpbrowser''),end'])
      mask Display: plot([-0.05, 1.05, NaN, -0.05, 1.05],[.01, .01, NaN, .99, .99])
  Zero_R : Constant  Description=|  Value=0  mask(TL_Constant){data={'date',734383.73415597226}}
      | Constant block of dSPACE TargetLink.
      | 
      | Output signal keeps the given constant value.
      settings: DeleteFcn=if exist('delete_tlblock','file')==2,delete_tlblock(gcbh);end  NameChangeFcn=if exist('rename_tlblock','file')==2,rename_tlblock(gcbh);end  OpenFcn=if exist('tl_open_blockdlg','file')==2,tl_open_blockdlg(gcbh);else,open_system(gcbh,'parameter');end
      mask Help: eval(['if exist(''tl_online_help'',''file'') == 2, tl_online_help(''Topic'',''TL_Constant''),else, web([''jar:file:///'',matlabroot,''/help/toolbox/simulink/help.jar!/slref/' lower(get_param(gcbh,'Blocktype')) '.html''], ''-helpbrowser''),end'])
      mask Display: plot([-0.05, 1.05, NaN, -0.05, 1.05],[.01, .01, NaN, .99, .99])
  Q : Outport  InitialOutput=0
  NOT_Q : Outport  Port=2  InitialOutput=0
  wires:
  LogOp_N/1 -> NOT_Q/1
  R/1 -> Switch_R/2
  Zero_R/1 -> Switch_R/1
  Switch_R/1 -> LogOp_N/1, Q/1, Memory_Q/1
  S/1 -> Switch_S/2
  One_S/1 -> Switch_S/1
  Switch_S/1 -> Switch_R/3
  Memory_Q/1 -> Switch_S/3

== system DAS/DEMO_FAS/DEMO_FAS/Subsystem/DEMO_FAS/DEMO_FAS_Funktion/Limiter/Limiter_Function/Limiter_Enabled/VERSION_INFO ==
  Copyright : Subsystem
      mask help: Copyright
      mask Display: disp('All copyrights by DaimlerChrysler');

== system DAS/DEMO_FAS/DEMO_FAS/Subsystem/DEMO_FAS/DEMO_FAS_Funktion/Limiter/Limiter_Function/Limiter_InitialSetValue/VERSION_INFO ==
  Copyright : Subsystem
      mask help: Copyright
      mask Display: disp('All copyrights by DaimlerChrysler');

== system DAS/DEMO_FAS/DEMO_FAS/Subsystem/DEMO_FAS/DEMO_FAS_Funktion/Limiter/Limiter_Function/Limiter_SetValue/VERSION_INFO ==
  Copyright : Subsystem
      mask help: Copyright
      mask Display: disp('All copyrights by DaimlerChrysler');

== system DAS/DEMO_FAS/DEMO_FAS/Subsystem/DEMO_FAS/DEMO_FAS_Funktion/Limiter/Limiter_Function/Limiter_SetValue/V_LimSetValueMinus ==
  V_LimiterSetValue : Inport
  Trigger : TriggerPort
  Data Store Write : DataStoreWrite  Description=|  DataStoreName=DEMO_FAS_V_LimiterSetValue  mask(TL_DataStoreWrite){data={'date',735342.5276524768}}
      | Data Store Write block of dSPACE TargetLink.
      | Use this block to specify outputs to global variables within the production code application.
      settings: DeleteFcn=if exist('delete_tlblock','file')==2,delete_tlblock(gcbh);end  NameChangeFcn=if exist('rename_tlblock','file')==2,rename_tlblock(gcbh);end  OpenFcn=if exist('tl_open_blockdlg','file')==2,tl_open_blockdlg(gcbh);else,open_system(gcbh,'parameter');end
      mask Help: eval(['if exist(''tl_online_help'',''file'') == 2, tl_online_help(''Topic'',''TL_DataStoreWrite''),else, web([''jar:file:///'',matlabroot,''/help/toolbox/simulink/help.jar!/slref/' lower(get_param(gcbh,'Blocktype')) '.html''], ''-helpbrowser''),end'])
      mask Display: plot([-0.05, 1.05, NaN, -0.05, 1.05],[.01, .01, NaN, .99, .99])
  Parameter : Constant  Description=|  Value=DEMO_FAS_Limiter_DELTA  SampleTime=-1  mask(TL_Constant){data={'output',{'variable','DEMO_FAS/p/Components/DEMO_FAS_CC_DELTA'},'date',735339.47752668976}}
      | Constant block of dSPACE TargetLink.
      | 
      | Output signal keeps the given constant value.
      settings: DeleteFcn=if exist('delete_tlblock','file')==2,delete_tlblock(gcbh);end  NameChangeFcn=if exist('rename_tlblock','file')==2,rename_tlblock(gcbh);end  OpenFcn=if exist('tl_open_blockdlg','file')==2,tl_open_blockdlg(gcbh);else,open_system(gcbh,'parameter');end
      mask Help: eval(['if exist(''tl_online_help'',''file'') == 2, tl_online_help(''Topic'',''TL_Constant''),else, web([''jar:file:///'',matlabroot,''/help/toolbox/simulink/help.jar!/slref/' lower(get_param(gcbh,'Blocktype')) '.html''], ''-helpbrowser''),end'])
      mask Display: plot([-0.05, 1.05, NaN, -0.05, 1.05],[.01, .01, NaN, .99, .99])
  Sum : Sum  Description=|  Inputs=+-  mask(TL_Sum){data={'logdata',{'plotchannels',[]},'date',735335.59140800929}}
      | Sum block of dSPACE TargetLink.
      | 
      | Output signal is equal to the sum of the input signals.
      | The list of signs is specified according to conventions for Simulink Sum blocks.
      settings: CopyFcn=if exist('tl_reset_reviewflag') == 2, tl_reset_reviewflag(gcbh); end  DeleteFcn=if exist('delete_tlblock','file')==2,delete_tlblock(gcbh);end  NameChangeFcn=if exist('rename_tlblock','file')==2,rename_tlblock(gcbh);end  OpenFcn=if exist('tl_open_blockdlg','file')==2,tl_open_blockdlg(gcbh);else,open_system(gcbh,'parameter');end
      mask Help: eval(['if exist(''tl_online_help'',''file'') == 2, tl_online_help(''Topic'',''TL_Sum''),else, web([''jar:file:///'',matlabroot,''/help/toolbox/simulink/help.jar!/slref/' lower(get_param(gcbh,'Blocktype')) '.html''], ''-helpbrowser''),end'])
      mask Display: plot([-0.05, 1.05, NaN, -0.05, 1.05],[.01, .01, NaN, .99, .99])
  VERSION_INFO : Subsystem  mask(VERSION_INFO_BLOCK){versinfo_data=struct('modname','DEMO_FAS/DEMO_FAS_Funktion/Limiter/Limiter_SetValue/V_LimSetValueMinus','version','1.1.1','date','18-Apr-2013','author','YVEDUHR','modtype',3,'variant',0,'remark',{{'~'}},'copyright',['Daimler AG'],'SGMLdescr','','prefix','','pfx_act',0,'ntselect',3,'asize',0), versinfo_string=Model: DEMO_FAS/DEMO_FAS_Funktion/Limiter/Limiter_SetValue/V_LimSetValueMinus\nVersion: 1.1.1\nDate: 18-Apr-2013\nAuthor: YVEDUHR\nModule: INTERNAL\n\nAll copyrights by Daimler AG}
      mask prompts: versinfo_data "Mask Parameter 1"; versinfo_string "Mask Parameter 2"
      mask help:
      | This is a Version Info Subsystem (empty)
      | All version Information is stored in Parameter "versinfo_data" and displayed
      settings: OpenFcn=edit_subsys_info('init')
      mask Display: disp(versinfo_string);
  wires:
  V_LimiterSetValue/1 -> Sum/1
  Parameter/1 -> Sum/2
  Sum/1 -> Data Store Write/1

== system DAS/DEMO_FAS/DEMO_FAS/Subsystem/DEMO_FAS/DEMO_FAS_Funktion/Limiter/Limiter_Function/Limiter_SetValue/V_LimSetValuePlus ==
  V_LimiterSetValue : Inport
  Trigger : TriggerPort
  Data Store Write : DataStoreWrite  Description=|  DataStoreName=DEMO_FAS_V_LimiterSetValue  mask(TL_DataStoreWrite){data={'date',735342.52752952545}}
      | Data Store Write block of dSPACE TargetLink.
      | Use this block to specify outputs to global variables within the production code application.
      settings: DeleteFcn=if exist('delete_tlblock','file')==2,delete_tlblock(gcbh);end  NameChangeFcn=if exist('rename_tlblock','file')==2,rename_tlblock(gcbh);end  OpenFcn=if exist('tl_open_blockdlg','file')==2,tl_open_blockdlg(gcbh);else,open_system(gcbh,'parameter');end
      mask Help: eval(['if exist(''tl_online_help'',''file'') == 2, tl_online_help(''Topic'',''TL_DataStoreWrite''),else, web([''jar:file:///'',matlabroot,''/help/toolbox/simulink/help.jar!/slref/' lower(get_param(gcbh,'Blocktype')) '.html''], ''-helpbrowser''),end'])
      mask Display: plot([-0.05, 1.05, NaN, -0.05, 1.05],[.01, .01, NaN, .99, .99])
  Parameter : Constant  Description=|  Value=DEMO_FAS_Limiter_DELTA  SampleTime=-1  mask(TL_Constant){data={'output',{'variable','DEMO_FAS/p/Components/DEMO_FAS_Limiter_DELTA'},'date',735339.47709418985}}
      | Constant block of dSPACE TargetLink.
      | 
      | Output signal keeps the given constant value.
      settings: DeleteFcn=if exist('delete_tlblock','file')==2,delete_tlblock(gcbh);end  NameChangeFcn=if exist('rename_tlblock','file')==2,rename_tlblock(gcbh);end  OpenFcn=if exist('tl_open_blockdlg','file')==2,tl_open_blockdlg(gcbh);else,open_system(gcbh,'parameter');end
      mask Help: eval(['if exist(''tl_online_help'',''file'') == 2, tl_online_help(''Topic'',''TL_Constant''),else, web([''jar:file:///'',matlabroot,''/help/toolbox/simulink/help.jar!/slref/' lower(get_param(gcbh,'Blocktype')) '.html''], ''-helpbrowser''),end'])
      mask Display: plot([-0.05, 1.05, NaN, -0.05, 1.05],[.01, .01, NaN, .99, .99])
  Sum : Sum  Description=|  mask(TL_Sum){data={'logdata',{'plotchannels',[]},'date',734383.73388289358}}
      | Sum block of dSPACE TargetLink.
      | 
      | Output signal is equal to the sum of the input signals.
      | The list of signs is specified according to conventions for Simulink Sum blocks.
      settings: CopyFcn=if exist('tl_reset_reviewflag') == 2, tl_reset_reviewflag(gcbh); end  DeleteFcn=if exist('delete_tlblock','file')==2,delete_tlblock(gcbh);end  NameChangeFcn=if exist('rename_tlblock','file')==2,rename_tlblock(gcbh);end  OpenFcn=if exist('tl_open_blockdlg','file')==2,tl_open_blockdlg(gcbh);else,open_system(gcbh,'parameter');end
      mask Help: eval(['if exist(''tl_online_help'',''file'') == 2, tl_online_help(''Topic'',''TL_Sum''),else, web([''jar:file:///'',matlabroot,''/help/toolbox/simulink/help.jar!/slref/' lower(get_param(gcbh,'Blocktype')) '.html''], ''-helpbrowser''),end'])
      mask Display: plot([-0.05, 1.05, NaN, -0.05, 1.05],[.01, .01, NaN, .99, .99])
  VERSION_INFO : Subsystem  mask(VERSION_INFO_BLOCK){versinfo_data=struct('modname','DEMO_FAS/DEMO_FAS_Funktion/Limiter/Limiter_SetValue/V_LimSetValuePlus','version','1.1.1','date','18-Apr-2013','author','YVEDUHR','modtype',3,'variant',0,'remark',{{'~'}},'copyright',['Daimler AG'],'SGMLdescr','','prefix','','pfx_act',0,'ntselect',3,'asize',0), versinfo_string=Model: DEMO_FAS/DEMO_FAS_Funktion/Limiter/Limiter_SetValue/V_LimSetValuePlus\nVersion: 1.1.1\nDate: 18-Apr-2013\nAuthor: YVEDUHR\nModule: INTERNAL\n\nAll copyrights by Daimler AG}
      mask prompts: versinfo_data "Mask Parameter 1"; versinfo_string "Mask Parameter 2"
      mask help:
      | This is a Version Info Subsystem (empty)
      | All version Information is stored in Parameter "versinfo_data" and displayed
      settings: OpenFcn=edit_subsys_info('init')
      mask Display: disp(versinfo_string);
  wires:
  V_LimiterSetValue/1 -> Sum/1
  Parameter/1 -> Sum/2
  Sum/1 -> Data Store Write/1

== system DAS/DEMO_FAS/DEMO_FAS/Subsystem/DEMO_FAS/DEMO_FAS_Funktion/Limiter/Limiter_Function/Limiter_StartUpSetValue/VERSION_INFO ==
  Copyright : Subsystem
      mask help: Copyright
      mask Display: disp('All copyrights by DaimlerChrysler');

== system DAS/DEMO_FAS/DEMO_FAS/Subsystem/DEMO_FAS/DEMO_FAS_Funktion/Limiter/Limiter_Function/VERSION_INFO/Copyright ==
